simulink model "simul4entrainement"  (R2023b)
settings: Solver=ode4  StartTime=0.0  StopTime=200  FixedStep=0.004  RelTol=1e-3
InitFcn:
  | start4_train
StopFcn:
  | stop4_train
values from neighbouring files (symbols this model uses):
  biais_acc = 0.003    [params4.m]    (also in start4.m)
undefined symbols (not defined in the file or in its folder): a_dlpf, b_dlpf
libraries: simulink x1, dspxfrm3 x1
settings Model: Creator=xavie  LastModifiedBy=xavie
settings DataIOCC: ReturnWorkspaceOutputs=off

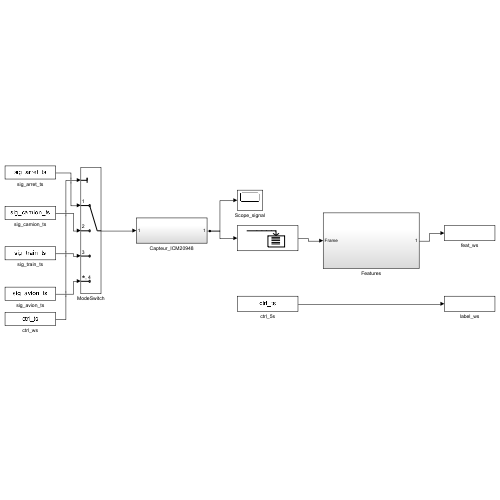
[thumbnail: Simulink's stored preview of the top-level diagram]
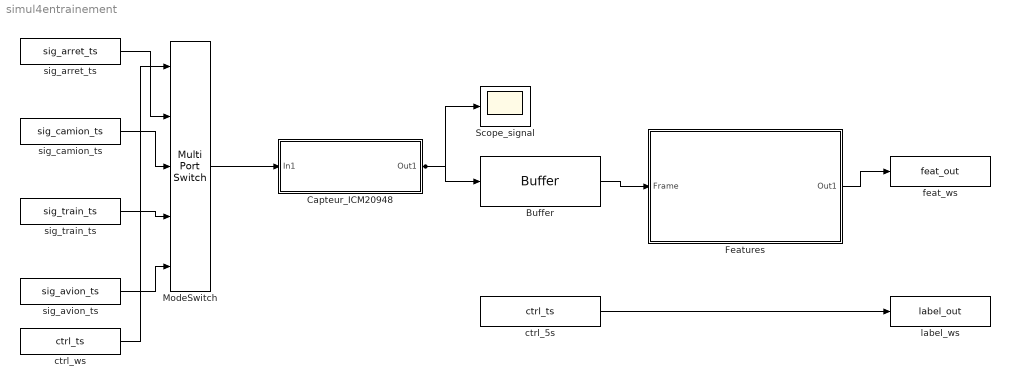
== system simul4entrainement ==
  Buffer : Buffer  N=2500  OverlapPercent=50
  Capteur_ICM20948 : Subsystem
  Features : Subsystem
  ModeSwitch : MultiPortSwitch  Inputs=4  SaturateOnIntegerOverflow=off  InputSameDT=off
  Scope_signal : Scope
  ctrl_5s : FromWorkspace  VariableName=ctrl_ts  SampleTime=10  Interpolate=off  OutputAfterFinalValue=Holding final value
  ctrl_ws : FromWorkspace  VariableName=ctrl_ts  SampleTime=0.004  Interpolate=off  OutputAfterFinalValue=Holding final value
  feat_ws : ToWorkspace  VariableName=feat_out  SampleTime=-1
  label_ws : ToWorkspace  VariableName=label_out  SampleTime=-1
  sig_arret_ts : FromWorkspace  VariableName=sig_arret_ts  SampleTime=0.004  Interpolate=off  OutputAfterFinalValue=Holding final value
  sig_avion_ts : FromWorkspace  VariableName=sig_avion_ts  SampleTime=0.004  Interpolate=off  OutputAfterFinalValue=Holding final value
  sig_camion_ts : FromWorkspace  VariableName=sig_camion_ts  SampleTime=0.004  Interpolate=off  OutputAfterFinalValue=Holding final value
  sig_train_ts : FromWorkspace  VariableName=sig_train_ts  SampleTime=0.004  Interpolate=off  OutputAfterFinalValue=Holding final value
  wires:
  ctrl_ws/1 -> ModeSwitch/1
  sig_arret_ts/1 -> ModeSwitch/2
  sig_camion_ts/1 -> ModeSwitch/3
  sig_train_ts/1 -> ModeSwitch/4
  sig_avion_ts/1 -> ModeSwitch/5
  ModeSwitch/1 -> Capteur_ICM20948/1(In1)
  Capteur_ICM20948/1(Out1) -> Scope_signal/1, Buffer/1
  Buffer/1 -> Features/1(Frame)
  Features/1(Out1) -> feat_ws/1
  ctrl_5s/1 -> label_ws/1

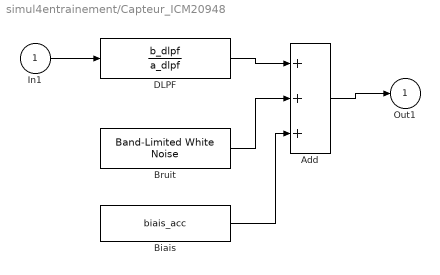
== system simul4entrainement/Capteur_ICM20948 ==
  In1 : Inport
  Add : Sum  Inputs=+++
  Biais : Constant  Value=biais_acc
  Bruit : simulink/Sources/Band-Limited White Noise  Cov=7.2e-09  Ts=0.004  seed=4321
  DLPF : DiscreteTransferFcn  Numerator=b_dlpf  Denominator=a_dlpf  SampleTime=0.004
  Out1 : Outport
  wires:
  In1/1 -> DLPF/1
  DLPF/1 -> Add/1
  Bruit/1 -> Add/2
  Biais/1 -> Add/3
  Add/1 -> Out1/1

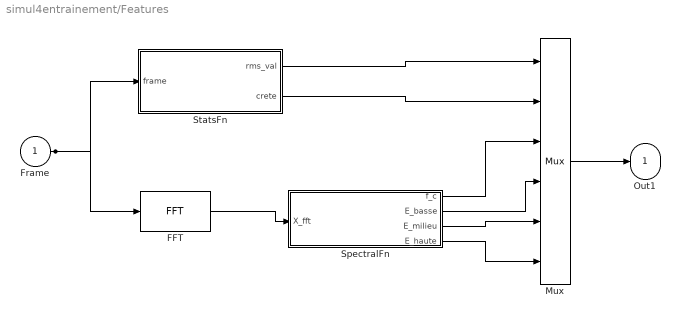
== system simul4entrainement/Features ==
  Frame : Inport
  FFT : dspxfrm3/FFT  FFTImplementation=Auto  CompMethod=Table lookup  TableOpt=NEW  TableOptActive=Speed  BitRevOrder=off  Normalize=off  InheritFFTLength=on  FFTLength=64  WrapInput=on  roundingMode=Floor  overflowMode=off  firstCoeffDataTypeStr=Inherit: Same word length as input  firstCoeffLastDataTypeStr=Inherit: Same word length as input  outputMin=[]  outputMax=[]
  Mux : Mux  Inputs=6
  SpectralFn : MATLAB Function  TreatAsAtomicUnit=on
  StatsFn : MATLAB Function  TreatAsAtomicUnit=on
  Out1 : Outport
  wires:
  Frame/1 -> FFT/1, StatsFn/1(frame)
  FFT/1 -> SpectralFn/1(X_fft)
  Mux/1 -> Out1/1
  StatsFn/1(rms_val) -> Mux/1
  StatsFn/2(crete) -> Mux/2
  SpectralFn/1(f_c) -> Mux/3
  SpectralFn/2(E_basse) -> Mux/4
  SpectralFn/3(E_milieu) -> Mux/5
  SpectralFn/4(E_haute) -> Mux/6

== matlab function simul4entrainement/Features/SpectralFn ==
  data: X_fft input; f_c output; E_basse output; E_milieu output; E_haute output
function [f_c, E_basse, E_milieu, E_haute] = spectral_fn(X_fft)
%SPECTRAL_FN  4 primitives spectrales a partir de la FFT brute d'une fenetre
%  Entree : X_fft   vecteur 2500x1 complexe — sortie directe du bloc FFT DSP
%  Sorties :
%    f_c      frequence centroide (Hz)
%    E_basse  energie relative bande [1-5 Hz]
%    E_milieu energie relative bande [5-50 Hz]
%    E_haute  energie relative bande [50-125 Hz]
%#codegen
fs_loc = 250;
N_loc  = 2500;

% DSP bilateral → spectre de puissance monolateral [1251 x 1]
X_pow  = abs(X_fft).^2 / (N_loc * fs_loc);
X_one  = X_pow(1:N_loc/2+1);
X_one(2:end-1) = 2 * X_one(2:end-1);    % doubler les termes internes

f_v    = (0:N_loc/2)' * fs_loc / N_loc; % vecteur frequences [0..125 Hz]
df_loc = fs_loc / N_loc;
E_tot  = sum(X_one) * df_loc + 1e-12;

f_c      = sum(f_v .* X_one) * df_loc / E_tot;
E_basse  = sum(X_one(f_v >= 1  & f_v <  5 )) * df_loc / E_tot;
E_milieu = sum(X_one(f_v >= 5  & f_v < 50 )) * df_loc / E_tot;
E_haute  = sum(X_one(f_v >= 50 & f_v < 125)) * df_loc / E_tot;
end

== matlab function simul4entrainement/Features/StatsFn ==
  data: frame input; rms_val output; crete output
function [rms_val, crete] = stats_fn(frame)
%STATS_FN  RMS et facteur de crete d'une fenetre temporelle
%  Entree : frame    vecteur 2500x1 (issu du bloc Buffer DSP)
%  Sorties :
%    rms_val  valeur efficace  sqrt(mean(x^2))
%    crete    facteur de crete max(|x|) / (rms + eps)
%#codegen
rms_val = sqrt(mean(frame.^2));
crete   = max(abs(frame)) / (rms_val + 1e-12);
end
